simulink library "lib_FaultDetection"  (R2017a)
settings: Solver=VariableStepAuto  StartTime=0.0  StopTime=10.0  RelTol=1e-3
undefined symbols (not defined in the file): cal, ENGTRQ_MSMCH_Degraded_CP, ENGTRQ_MSMCH_ErrCritical_CP, ENGTRQ_MSMCH_LimpHome_CP
libraries: simulink x57, Diagnostic x4, lib_SystemDiag x1
(part 1 of 3)
settings Model: Creator=Di Russo  LastModifiedBy=Di Russo

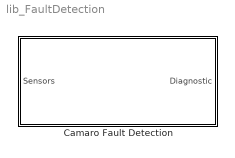
== system lib_FaultDetection ==
  Camaro Fault Detection : Subsystem

== system lib_FaultDetection/Camaro Fault Detection ==
  Sensors : Inport
  Component Diagnostic : Subsystem
  Input Conversions : Subsystem
  Signal Diagnostic : Subsystem
  SystemDiag : lib_SystemDiag/SystemDiag
  Diagnostic : Outport
  wires:
  SystemDiag/1 -> Diagnostic/1
  Sensors/1 -> Input Conversions/1(RawSig)
  Input Conversions/1(VehSig) -> Signal Diagnostic/1(VehSig)
  Component Diagnostic/1(CompDiag) -> SystemDiag/1
  Signal Diagnostic/1(SignalDiag) -> Component Diagnostic/1(SignalDiag)

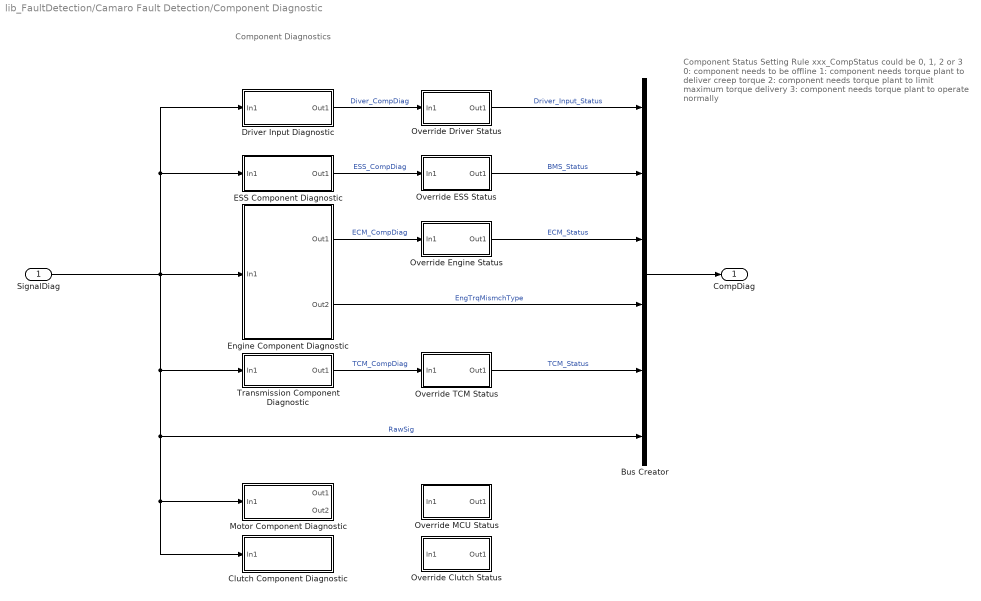
== system lib_FaultDetection/Camaro Fault Detection/Component Diagnostic ==
  note: Component Diagnostics
  note: Component Status Setting Rule
      | xxx_CompStatus could be 0, 1, 2 or 3
      | 0: component needs to be offline
      | 1: component needs torque plant to deliver creep torque
      | 2: component needs torque plant to limit maximum torque delivery
      | 3: component needs torque plant to operate normally
  SignalDiag : Inport
  Bus Creator : BusCreator  Inputs=6
  Clutch Component Diagnostic : Subsystem
  Driver Input Diagnostic : Subsystem
  ESS Component Diagnostic : Subsystem
  Engine Component Diagnostic : Subsystem
  Motor Component Diagnostic : Subsystem
  Override Clutch Status : Subsystem
  Override Driver Status : Subsystem
  Override ESS Status : Subsystem
  Override Engine Status : Subsystem
  Override MCU Status : Subsystem
  Override TCM Status : Subsystem
  Transmission Component Diagnostic : Subsystem
  CompDiag : Outport
  wires:
  Engine Component Diagnostic/2(Out2) -> Bus Creator/4  "EngTrqMismchType"
  Override Driver Status/1(Out1) -> Bus Creator/1  "Driver_Input_Status"
  Override TCM Status/1(Out1) -> Bus Creator/5  "TCM_Status"
  Override Engine Status/1(Out1) -> Bus Creator/3  "ECM_Status"
  Override ESS Status/1(Out1) -> Bus Creator/2  "BMS_Status"
  Transmission Component Diagnostic/1(Out1) -> Override TCM Status/1(In1)  "TCM_CompDiag"
  Engine Component Diagnostic/1(Out1) -> Override Engine Status/1(In1)  "ECM_CompDiag"
  ESS Component Diagnostic/1(Out1) -> Override ESS Status/1(In1)  "ESS_CompDiag"
  Driver Input Diagnostic/1(Out1) -> Override Driver Status/1(In1)  "Diver_CompDiag"
  Bus Creator/1 -> CompDiag/1
  SignalDiag/1 -> Driver Input Diagnostic/1(In1), ESS Component Diagnostic/1(In1), Bus Creator/6, Motor Component Diagnostic/1(In1), Clutch Component Diagnostic/1(In1), Transmission Component Diagnostic/1(In1), Engine Component Diagnostic/1(In1)  "RawSig"

== system lib_FaultDetection/Camaro Fault Detection/Input Conversions ==
  note: These subsystems convert variable types to match those used in the
      | supervisor. In addition, override switches installed on each signal can
      | be used to manually override and signal for testing purposes
  note: Input Conversions and Override Switches
  RawSig : Inport
  BMS_Conversions : Subsystem
  Bus Creator : BusCreator  Inputs=6
  Clutch_Conversions : Subsystem
  DriverInput_Conversions : Subsystem
  ECM_Conversions : Subsystem
  MCU_Conversions : Subsystem
  TCM_Conversions : Subsystem
  VehSig : Outport
  wires:
  TCM_Conversions/1(Out1) -> Bus Creator/4
  ECM_Conversions/1(Out1) -> Bus Creator/3
  RawSig/1 -> Clutch_Conversions/1(Sensors), Bus Creator/6, TCM_Conversions/1(In1), ECM_Conversions/1(In1), BMS_Conversions/1(In1), DriverInput_Conversions/1(In1)  "RawSig"
  BMS_Conversions/1(Out1) -> Bus Creator/2
  Bus Creator/1 -> VehSig/1  "InputConvAndOvrd"
  DriverInput_Conversions/1(Out1) -> Bus Creator/1
  Clutch_Conversions/1(Out1) -> Bus Creator/5

== system lib_FaultDetection/Camaro Fault Detection/Signal Diagnostic ==
  note: Signal Diagnostics
  note: These subsystems evaluate each signal for proper value range and other checks
  VehSig : Inport
  Bus Creator : BusCreator  Inputs=7
  Clutch Signal Diagnostic : Subsystem
  Driver Signal Diagnostic : Subsystem
  ESS Signal Diagnostic : Subsystem
  Engine Signal Diagnostic : Subsystem
  Motor Signal Diagnostic : Subsystem
  Subsystem1 : Subsystem
      mask Display: fprintf('Signal Naming Rule')
  Transmission Signal Diagnostic : Subsystem
  SignalDiag : Outport
  wires:
  Bus Creator/1 -> SignalDiag/1  "SignalDiag"
  Transmission Signal Diagnostic/1(Transmission_SigDiag) -> Bus Creator/5  "Transmission_SigDiag"
  Engine Signal Diagnostic/1(Engine_SigDiag) -> Bus Creator/4  "Engine_SigDiag"
  ESS Signal Diagnostic/1(ESS_SigDiag) -> Bus Creator/2  "ESS_SigDiag"
  Driver Signal Diagnostic/1(Driver_SigDiag) -> Bus Creator/1  "Driver_SigDiag"
  VehSig/1 -> Driver Signal Diagnostic/1(Sensors1), ESS Signal Diagnostic/1(Sensors1), Motor Signal Diagnostic/1(Sensors1), Engine Signal Diagnostic/1(Sensors1), Transmission Signal Diagnostic/1(Sensors1), Bus Creator/7, Clutch Signal Diagnostic/1(Sensors1)
  Clutch Signal Diagnostic/1(Out2) -> Bus Creator/6  "Clutch_SigDiag"
  Motor Signal Diagnostic/1(Motor_SigDiag) -> Bus Creator/3  "Motor_SigDiag"

== system lib_FaultDetection/Camaro Fault Detection/Component Diagnostic/Clutch Component Diagnostic ==
  note: 0: component Offline
      | 1: component Online
  In1 : Inport
  Bus Selector : BusSelector  OutputSignals=Motor_SigDiag.MCURollingAliveActive,Motor_SigDiag.MCUTemp_degC_SigValid,Motor_SigDiag.MotorTemp_degC_SigValid,Motor_SigDiag.Motor_TrqCmd_Nm_SigValid,Motor_SigDiag.Torq_Feedback_Nm_SigValid,Motor_SigDiag.MCUTrqCmd_Nm,Motor_SigDiag.Torq_Feedback_Nm,Motor_SigDiag.Motor_Speed_rpm_SigValid,Motor_SigDiag.MCUTempRange[0_4],Motor_SigDiag.MotorTempRange[0_4],Motor_SigDiag.Direction_Command_SigValid,Motor_SigDiag.Direction_feedback_SigValid,Motor_SigDiag.Inverter_enable_state_SigValid,Motor_SigDiag.Direction_Command_0_1,Motor_SigDiag.Direction_feedback_0_1,Motor_SigDiag.Inverter_enable_state_0_1,Motor_SigDiag.DC_Bus_Voltage_SigValid,Motor_SigDiag.DC_Bus_Voltage_V,ESS_SigDiag.hvBattVolt_V
  wires:
  In1/1 -> Bus Selector/1

== system lib_FaultDetection/Camaro Fault Detection/Component Diagnostic/Driver Input Diagnostic ==
  note: APP1
      | APP2
      | BPP
      | Driver Component Status
      |
      | 1
      | 1
      | 1
      | 1
      |
      | 0
      | 1
      | 1
      | 1
      |
      | 1
      | 0
      | 1
      | 1
      |
      | 0
      | 0
      | 1
      | 0
      |
      | 1
      | 1
      | 0
      | 0
      |
      | 0
      | 0
      | 0
      | 0
  note: Driver_CompStatus
      | 1 = Component Online
      | 0 = Component Offline
  In1 : Inport
  Bus Selector : BusSelector  OutputSignals=Driver_SigDiag.Drv_APP1_[%]_SigValid,Driver_SigDiag.Drv_APP2_[%]_SigValid,Driver_SigDiag.Drv_APP_Agree,Driver_SigDiag.Drv_BPP_[%]_SigValid,Driver_SigDiag.Drv_KeyPos_[0 3]_SigValid,Driver_SigDiag.Drv_PRNDL_SigValid,Driver_SigDiag.Brake_Failed
  Driver_Input_Diag : Stateflow chart  TreatAsAtomicUnit=on
  Logical Operator : Logic  Inputs=3  AllPortsSameDT=off  OutDataTypeStr=boolean
  Out1 : Outport
  wires:
  Bus Selector/7 -> Driver_Input_Diag/5(BrakeFail)  "<Brake_Failed>"
  Bus Selector/6 -> Driver_Input_Diag/4(PRNDL)  "<Drv_PRNDL_SigValid>"
  Bus Selector/5 -> Driver_Input_Diag/3(KeyPos)  "<Drv_KeyPos_[0 3]_SigValid>"
  Bus Selector/3 -> Logical Operator/3  "<Drv_APP_Agree>"
  Logical Operator/1 -> Driver_Input_Diag/1(APP_Valid)  "APP_Valid"
  Driver_Input_Diag/1(Driver_Input_Status) -> Out1/1  "Driver_Input_Status"
  Bus Selector/4 -> Driver_Input_Diag/2(Drv_BPP_SigValid)  "<Drv_BPP_[%]_SigValid>"
  Bus Selector/2 -> Logical Operator/2  "<Drv_APP2_[%]_SigValid>"
  Bus Selector/1 -> Logical Operator/1  "<Drv_APP1_[%]_SigValid>"
  In1/1 -> Bus Selector/1

== system lib_FaultDetection/Camaro Fault Detection/Component Diagnostic/ESS Component Diagnostic ==
  note: (Need modify)
  In1 : Inport
  BMS_CompDiag1 : Stateflow chart  TreatAsAtomicUnit=on
  Bus Selector : BusSelector  OutputSignals=ESS_SigDiag.BMS_RollingAliveActive_SigValid,ESS_SigDiag.BMS_contactorsFailed_Detected,ESS_SigDiag.BMS_essTemp_[degC]_SigValid,ESS_SigDiag.essTempRange[0_4],ESS_SigDiag.BMS_essSOC_0_1_SigValid,ESS_SigDiag.essTempRange[0_4],ESS_SigDiag.essCur_A_SigValid,ESS_SigDiag.BMSgdf_SigValid,Driver_SigDiag.Drv_KeyPos_[0 3]_SigValid
  Compare To Zero : simulink/Logic and Bit Operations/Compare To Zero  relop===  OutDataTypeStr=boolean
  Data Type Conversion : DataTypeConversion
  HVessFltReset : Constant
  Logical Operator : Logic  Operator=OR  AllPortsSameDT=off  OutDataTypeStr=boolean
  Logical Operator1 : Logic  AllPortsSameDT=off  OutDataTypeStr=boolean
  Terminator : Terminator
  Terminator1 : Terminator
  Out1 : Outport
  wires:
  [contactorsFailed_Detected] -> Logical Operator1/1
  Logical Operator1/1 -> BMS_CompDiag1/6(ess_GroundFault)
  Bus Selector/8 -> Logical Operator1/2  "<BMSgdf_SigValid>"
  Logical Operator/1 -> BMS_CompDiag1/7(ClearFault)
  HVessFltReset/1 -> Logical Operator/2
  Compare To Zero/1 -> Logical Operator/1
  Bus Selector/9 -> Compare To Zero/1  "<Drv_KeyPos_[0 3]_SigValid>"
  Bus Selector/7 -> BMS_CompDiag1/5(essCur_A_SigValid)  "<essCur_A_SigValid>"
  Bus Selector/6 -> Terminator1/1  "<essTempRange[0_4]>"
  Bus Selector/5 -> BMS_CompDiag1/4(BMS_essSOC_0_1_SigValid)  "<BMS_essSOC_0_1_SigValid>"
  Data Type Conversion/1 -> BMS_CompDiag1/3(BMS_essTemp_SigValid)  "BMS_essTemp_SigValid"
  Bus Selector/3 -> Data Type Conversion/1  "<BMS_essTemp_[degC]_SigValid>"
  Bus Selector/4 -> Terminator/1  "<essTempRange[0_4]>"
  BMS_CompDiag1/1(BMS_Status) -> Out1/1  "BMS_Status"
  Bus Selector/2 -> BMS_CompDiag1/2(BMS_contactorsFailed_SigValid), [contactorsFailed_Detected]  "<BMS_contactorsFailed_Detected>"
  Bus Selector/1 -> BMS_CompDiag1/1(BMS_RollingAliveActive_SigValid)  "<BMS_RollingAliveActive_SigValid>"
  In1/1 -> Bus Selector/1

== system lib_FaultDetection/Camaro Fault Detection/Component Diagnostic/Engine Component Diagnostic ==
  note: Notes
  note: 0: component needs to be offline
      | 1: component needs torque plant to deliver creep torque
      | 2: component needs torque plant to limit maximum torque delivery
      | 3: component needs torque plant to operate normally
  note: add the temperature, mismatch torquesignal and have different status to the component
  note: Eng_tempRange
      | 1: normal
      | 2: high range
      | 3:above max
  note: ENGTRQ_MSMCH_Degraded_CP (40Nm): ENGTRQ_Degraded fault code.
      | ENGTRQ_MSMCH_LimpHome_CP (70Nm): ENGTRQ_LimpHome
      | ENGTRQ_MSMCH_ErrCritical_CP (100Nm): ENGTRQ_ErrCritical
  note: Eng_Torq_MsmchLevel
      | 1:Normal torque
      | 2: Limit max power
      | 3: Deliver creep torque
      | 4: offline
  In1 : Inport
  Bus Selector : BusSelector  OutputSignals=Engine_SigDiag.ECMRollingAliveActive,Engine_SigDiag.engTrqCmdRecvd_SigValid,Engine_SigDiag.ECMTrqCmd_Nm,Engine_SigDiag.EngActStdyStTorq_Nm,Engine_SigDiag.EngRunAtValid,Engine_SigDiag.Engine_Speed_rpm_SigValid,Engine_SigDiag.Eng_TempValid,Engine_SigDiag.Eng_TempRange[123],Driver_SigDiag.Drv_KeyPos_[0 3]_SigValid
  Bus Selector1 : BusSelector  OutputSignals=Eng_Torque_Mismch_Critical
  Compare To Zero : simulink/Logic and Bit Operations/Compare To Zero  relop===  OutDataTypeStr=boolean
  ECM_CompDiag : Stateflow chart  TreatAsAtomicUnit=on
  Eng_FltReset : Constant
  Eng_Torq_MsmchLevel : Stateflow chart  Commented=on  TreatAsAtomicUnit=on
  Logical Operator : Logic  Operator=OR  AllPortsSameDT=off  OutDataTypeStr=boolean
  Override  engTrqCmd : Subsystem
  Terminator1 : Terminator
  TorqMismatch Detection : Subsystem
  Out1 : Outport
  Out2 : Outport  Port=2
  wires:
  Override  engTrqCmd/1(Out1) -> ECM_CompDiag/2(engTrqCmdRecvd_SigValid)
  Bus Selector1/1 -> ECM_CompDiag/3(Eng_Torq_Msmch)  "<Eng_Torque_Mismch_Critical>"
  TorqMismatch Detection/1(Eng_Torque_Mismch) -> Out2/1, Bus Selector1/1  "EngTrqMismchType"
  Bus Selector/5 -> TorqMismatch Detection/3(In3)  "<EngRunAtValid>"
  Bus Selector/4 -> TorqMismatch Detection/2(In2)  "<EngActStdyStTorq_Nm>"
  Bus Selector/3 -> TorqMismatch Detection/1(In1)  "<ECMTrqCmd_Nm>"
  Bus Selector/8 -> ECM_CompDiag/5(Eng_TempRange_123)  "<Eng_TempRange[123]>"
  Bus Selector/7 -> Terminator1/1  "<Eng_TempValid>"
  Bus Selector/9 -> Compare To Zero/1  "<Drv_KeyPos_[0 3]_SigValid>"
  Logical Operator/1 -> ECM_CompDiag/6(ClearFault)
  Eng_FltReset/1 -> Logical Operator/2
  Compare To Zero/1 -> Logical Operator/1
  ECM_CompDiag/1(ECM_Status) -> Out1/1  "ECM_Status"
  Bus Selector/6 -> ECM_CompDiag/4(Engine_Speed_rpm_SigValid)  "<Engine_Speed_rpm_SigValid>"
  Bus Selector/2 -> Override  engTrqCmd/1(In1)  "<engTrqCmdRecvd_SigValid>"
  Bus Selector/1 -> ECM_CompDiag/1(ECM_RollingAliveActive)  "<ECMRollingAliveActive>"
  In1/1 -> Bus Selector/1

== system lib_FaultDetection/Camaro Fault Detection/Component Diagnostic/Motor Component Diagnostic ==
  note: 0: component needs to be offline
      | 1: component needs torque plant to deliver creep torque
      | 2: component needs torque plant to limit maximum torque delivery
      | 3: component needs torque plant to operate normally
  In1 : Inport
  Bus Creator : BusCreator  Inputs=1
  Bus Selector : BusSelector  OutputSignals=Motor_SigDiag.MCURollingAliveActive,Motor_SigDiag.MCUTemp_degC_SigValid,Motor_SigDiag.MotorTemp_degC_SigValid,Motor_SigDiag.Motor_TrqCmd_Nm_SigValid,Motor_SigDiag.Torq_Feedback_Nm_SigValid,Motor_SigDiag.MCUTrqCmd_Nm,Motor_SigDiag.Torq_Feedback_Nm,Motor_SigDiag.Motor_Speed_rpm_SigValid,Motor_SigDiag.MCUTempRange[0_4],Motor_SigDiag.MotorTempRange[0_4],Motor_SigDiag.Direction_Command_SigValid,Motor_SigDiag.Direction_feedback_SigValid,Motor_SigDiag.Inverter_enable_state_SigValid,Motor_SigDiag.Direction_Command_0_1,Motor_SigDiag.Direction_feedback_0_1,Motor_SigDiag.Inverter_enable_state_0_1,Motor_SigDiag.DC_Bus_Voltage_SigValid,Motor_SigDiag.DC_Bus_Voltage_V,ESS_SigDiag.hvBattVolt_V
  Bus Selector1 : BusSelector  OutputSignals=MCU_Torque_Mismch_Critical
  MCU_CompDiag : Stateflow chart  TreatAsAtomicUnit=on
  MCU_ESS_Voltage_Mismatch : Subsystem
  Motor_Direction_Mismatch : Subsystem
  Override  fault : Subsystem
  Override  fault1 : Subsystem
  Terminator1 : Terminator
  Torque_Mismatch : Subsystem
  Out1 : Outport
  Out2 : Outport  Port=2
  wires:
  In1/1 -> Bus Selector/1
  MCU_CompDiag/1(MCU_Status) -> Bus Creator/1  "MCU_Status"
  Bus Selector/1 -> MCU_CompDiag/1(MCU_RollingAliveActive)  "<MCURollingAliveActive>"
  Bus Selector/2 -> MCU_CompDiag/2(MCUTemp_degC_SigValid)  "<MCUTemp_degC_SigValid>"
  Bus Selector/3 -> MCU_CompDiag/3(MotorTemp_degC_SigValid)  "<MotorTemp_degC_SigValid>"
  Bus Selector/4 -> MCU_CompDiag/4(Motor_TrqCmd_Nm_SigValid)  "<Motor_TrqCmd_Nm_SigValid>"
  Bus Selector/8 -> MCU_CompDiag/7(Motor_Speed_rpm_SigValid)  "<Motor_Speed_rpm_SigValid>"
  Bus Selector/9 -> MCU_CompDiag/8(MCUTempRange)  "<MCUTempRange[0_4]>"
  Bus Creator/1 -> Out1/1
  Bus Selector/13 -> Terminator1/1  "<Inverter_enable_state_SigValid>"
  Bus Selector/6 -> Torque_Mismatch/1(MCU_torq_command)  "<MCUTrqCmd_Nm>"
  Bus Selector/7 -> Torque_Mismatch/2(Torq_feedback)  "<Torq_Feedback_Nm>"
  Bus Selector/14 -> Motor_Direction_Mismatch/1(Direction_Command)  "<Direction_Command_0_1>"
  Bus Selector/15 -> Motor_Direction_Mismatch/2(Direction_Feedback)  "<Direction_feedback_0_1>"
  Bus Selector/16 -> Motor_Direction_Mismatch/3(Inverter_enable_state)  "<Inverter_enable_state_0_1>"
  Bus Selector/11 -> MCU_CompDiag/10(Dir_Command_SigValid)  "<Direction_Command_SigValid>"
  Bus Selector/12 -> MCU_CompDiag/11(Dir_feedback_SigValid)  "<Direction_feedback_SigValid>"
  Bus Selector/5 -> MCU_CompDiag/5(Torq_Feedback_SigValid)  "<Torq_Feedback_Nm_SigValid>"
  Bus Selector/17 -> MCU_CompDiag/13(dc_bus_voltage_SigValid)  "<DC_Bus_Voltage_SigValid>"
  Bus Selector/18 -> MCU_ESS_Voltage_Mismatch/1(MCU_Voltage)  "<DC_Bus_Voltage_V>"
  Bus Selector/19 -> MCU_ESS_Voltage_Mismatch/2(ESS_Voltage)  "< hvBattVolt_V>"
  MCU_ESS_Voltage_Mismatch/1(MCU_ESS_Voltage_Mismch) -> Override  fault/1(In1)
  Motor_Direction_Mismatch/1(Direction_Mismch) -> Override  fault1/1(In1)
  Torque_Mismatch/1(MCU_Torque_Mismch) -> Bus Selector1/1, Out2/1  "MCU_Torque_Mismch"
  Bus Selector1/1 -> MCU_CompDiag/6(MCU_torq_mismch)  "<MCU_Torque_Mismch_Critical>"
  Override  fault/1(Out1) -> MCU_CompDiag/14(Voltage_Mismch)
  Override  fault1/1(Out1) -> MCU_CompDiag/12(Dir_Mismch)
  Bus Selector/10 -> MCU_CompDiag/9(MotTempRange)  "<MotorTempRange[0_4]>"

== system lib_FaultDetection/Camaro Fault Detection/Component Diagnostic/Override Clutch Status ==
  note: Override Switch Subsystem
  note: This subsystem is used to override the model value of a signal to a constant value
  In1 : Inport
  Multiport Switch : MultiPortSwitch  DataPortOrder=Zero-based contiguous  Inputs=2  zeroidx=on
  Override Value : Constant  Value=2  OutDataTypeStr=double
  Signal Override Switch 0 = Use Model 1 = Use Constant : Constant  Value=0
  Out1 : Outport
  wires:
  Override Value/1 -> Multiport Switch/3
  Multiport Switch/1 -> Out1/1
  In1/1 -> Multiport Switch/2
  Signal Override Switch 0 = Use Model 1 = Use Constant/1 -> Multiport Switch/1

== system lib_FaultDetection/Camaro Fault Detection/Component Diagnostic/Override Driver Status ==
  note: Override Switch Subsystem
  note: This subsystem is used to override the model value of a signal to a constant value
  In1 : Inport
  Data Type Conversion3 : DataTypeConversion
  Override Value : Constant  OutDataTypeStr=double
  Override_Driver_Status : Constant  Value=0
  Switch : Switch  Criteria=u2 > Threshold
  Out1 : Outport
  wires:
  Data Type Conversion3/1 -> Switch/3
  Override Value/1 -> Switch/1
  Switch/1 -> Out1/1
  In1/1 -> Data Type Conversion3/1
  Override_Driver_Status/1 -> Switch/2

== system lib_FaultDetection/Camaro Fault Detection/Component Diagnostic/Override ESS Status ==
  note: Override Switch Subsystem
  note: This subsystem is used to override the model value of a signal to a constant value
  In1 : Inport
  Data Type Conversion3 : DataTypeConversion
  Override Value : Constant  Value=2  OutDataTypeStr=double
  Override_ESS_Status : Constant  Value=0
  Switch : Switch  Criteria=u2 > Threshold
  Terminator : Terminator
  Out1 : Outport
  wires:
  Data Type Conversion3/1 -> Switch/3
  Override Value/1 -> Switch/1, Out1/1
  Override_ESS_Status/1 -> Switch/2
  In1/1 -> Data Type Conversion3/1
  Switch/1 -> Terminator/1

== system lib_FaultDetection/Camaro Fault Detection/Component Diagnostic/Override Engine Status ==
  note: Override Switch Subsystem
  note: This subsystem is used to override the model value of a signal to a constant value
  In1 : Inport
  Data Type Conversion3 : DataTypeConversion
  Override Value1 : Constant  Value=2  OutDataTypeStr=double
  Override_Engine_Status : Constant  Value=0
  Switch : Switch  Criteria=u2 > Threshold
  Terminator : Terminator
  Out1 : Outport
  wires:
  Data Type Conversion3/1 -> Switch/3
  Override_Engine_Status/1 -> Switch/2
  Override Value1/1 -> Switch/1, Out1/1
  In1/1 -> Data Type Conversion3/1
  Switch/1 -> Terminator/1

== system lib_FaultDetection/Camaro Fault Detection/Component Diagnostic/Override MCU Status ==
  note: This subsystem is used to override the model value of a signal to a constant value
  note: Override Switch Subsystem
  In1 : Inport
  Multiport Switch : MultiPortSwitch  DataPortOrder=Zero-based contiguous  Inputs=2  zeroidx=on
  Override Value : Constant  Value=2  OutDataTypeStr=double
  Signal Override Switch 0 = Use Model 1 = Use Constant : Constant  Value=0
  Out1 : Outport
  wires:
  Signal Override Switch 0 = Use Model 1 = Use Constant/1 -> Multiport Switch/1
  In1/1 -> Multiport Switch/2
  Multiport Switch/1 -> Out1/1
  Override Value/1 -> Multiport Switch/3

== system lib_FaultDetection/Camaro Fault Detection/Component Diagnostic/Override TCM Status ==
  note: Override Switch Subsystem
  note: This subsystem is used to override the model value of a signal to a constant value
  In1 : Inport
  Data Type Conversion3 : DataTypeConversion
  Override Value1 : Constant  Value=2  OutDataTypeStr=double
  Override_TCM_Status : Constant  Value=0
  Switch : Switch  Criteria=u2 > Threshold
  Out1 : Outport
  wires:
  Data Type Conversion3/1 -> Switch/3
  Override Value1/1 -> Switch/1
  Override_TCM_Status/1 -> Switch/2
  Switch/1 -> Out1/1
  In1/1 -> Data Type Conversion3/1

== system lib_FaultDetection/Camaro Fault Detection/Component Diagnostic/Transmission Component Diagnostic ==
  In1 : Inport
  Bus Selector : BusSelector  OutputSignals=Transmission_SigDiag.TCMRollingAliveActive_SigValid,Transmission_SigDiag.LvrPosTrnsShft_SigValid,Transmission_SigDiag.TransEstGear_SigValid,Transmission_SigDiag.LockupCmd_SigValid,Transmission_SigDiag.VehDirFault
  TCM_CompDia : Stateflow chart  TreatAsAtomicUnit=on
  Out1 : Outport
  wires:
  Bus Selector/5 -> TCM_CompDia/5(VehDirFault)  "<VehDirFault>"
  TCM_CompDia/1(TCM_Status) -> Out1/1  "TCM_Status"
  Bus Selector/4 -> TCM_CompDia/4(LockupCmd_SigValid)  "<LockupCmd_SigValid>"
  Bus Selector/3 -> TCM_CompDia/3(TransEstGear_SigValid)  "<TransEstGear_SigValid>"
  Bus Selector/2 -> TCM_CompDia/2(LvrPosTrnsShft_SigValid)  "<LvrPosTrnsShft_SigValid>"
  Bus Selector/1 -> TCM_CompDia/1(TCMRollingAliveActive_SigValid)  "<TCMRollingAliveActive_SigValid>"
  In1/1 -> Bus Selector/1

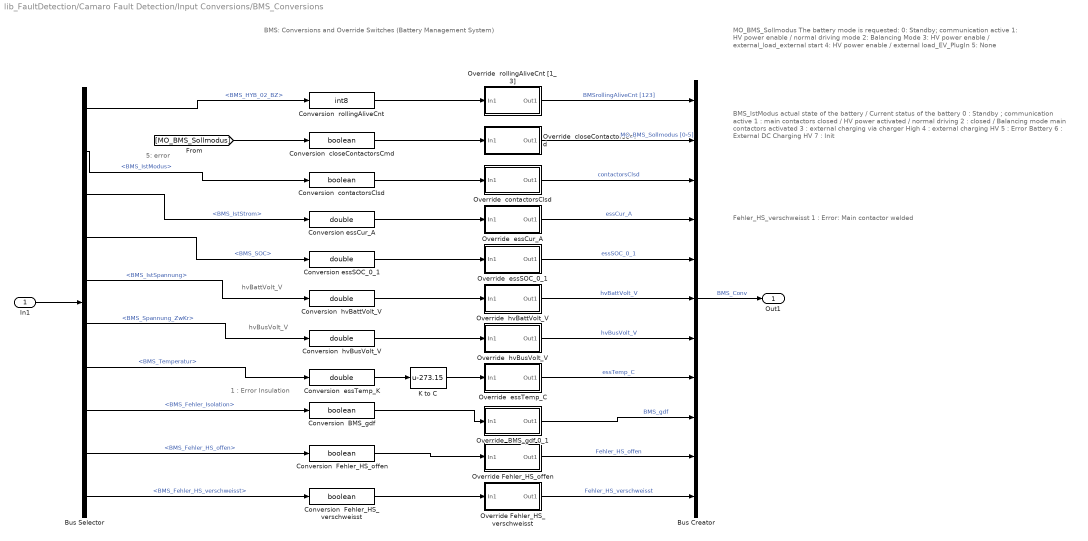
== system lib_FaultDetection/Camaro Fault Detection/Input Conversions/BMS_Conversions ==
  note: BMS: Conversions and Override Switches
      | (Battery Management System)
  note: hvBattVolt_V
  note: hvBusVolt_V
  note: 5: error
  note: 1 : Error Insulation
  note: MO_BMS_Sollmodus
      | The battery mode is requested:
      | 0: Standby; communication active
      | 1: HV power enable / normal driving mode
      | 2: Balancing Mode
      | 3: HV power enable / external_load_external start
      | 4: HV power enable / external load_EV_PlugIn
      | 5: None
  note: BMS_IstModus
      | actual state of the battery / Current status of the battery
      | 0 : Standby ; communication active
      | 1 : main contactors closed / HV power activated / normal driving
      | 2 : closed / Balancing mode main contactors activated
      | 3 : external charging via charger High
      | 4 : external charging HV
      | 5 : Error Battery
      | 6 : External DC Charging HV
      | 7 : Init
  note: Fehler_HS_verschweisst
      | 1 : Error: Main contactor welded
  In1 : Inport
  Bus Creator : BusCreator  Inputs=11
  Bus Selector : BusSelector  OutputSignals=from_CAN.fromHV_CAN.from_BMSHybrid.BMS_HYB_02.BMS_HYB_02_BZ,from_CAN.fromHV_CAN.from_BMSHybrid.BMS_HYB_02.BMS_IstModus,from_CAN.fromHV_CAN.from_BMSHybrid.BMS_HYB_02.BMS_IstStrom,from_CAN.fromHV_CAN.from_BMSHybrid.BMS_SOC,from_CAN.fromHV_CAN.from_BMSHybrid.BMS_HYB_02.BMS_IstSpannung,from_CAN.fromHV_CAN.from_BMSHybrid.BMS_Spannung_ZwKr,from_CAN.fromHV_CAN.from_BMSHybrid.BMS_Temperatur,from_CAN.fromHV_CAN.from_BMSHybrid.BMS_Fehler_Isolation,from_CAN.fromHV_CAN.from_BMSHybrid.BMS_HYB_02.BMS_Fehler_HS_offen,from_CAN.fromHV_CAN.from_BMSHybrid.BMS_Fehler_HS_verschweisst
  Conversion  BMS_gdf : DataTypeConversion  OutDataTypeStr=boolean
  Conversion  Fehler_HS_offen : DataTypeConversion  OutDataTypeStr=boolean
  Conversion  Fehler_HS_verschweisst : DataTypeConversion  OutDataTypeStr=boolean
  Conversion  closeContactorsCmd : DataTypeConversion  OutDataTypeStr=boolean
  Conversion  contactorsClsd : DataTypeConversion  OutDataTypeStr=boolean
  Conversion  essTemp_K : DataTypeConversion  OutDataTypeStr=double
  Conversion  hvBattVolt_V : DataTypeConversion  OutDataTypeStr=double
  Conversion  hvBusVolt_V : DataTypeConversion  OutDataTypeStr=double
  Conversion  rollingAliveCnt : DataTypeConversion  OutDataTypeStr=int8
  Conversion essCur_A : DataTypeConversion  OutDataTypeStr=double
  Conversion essSOC_0_1 : DataTypeConversion  OutDataTypeStr=double
  K to C : Bias  Bias=-273.15
  Override  BMS_gdf 0_1 : Subsystem
  Override  closeContactorsCmd : Subsystem
  Override  contactorsClsd : Subsystem
  Override  essCur_A : Subsystem
  Override  essSOC_0_1 : Subsystem
  Override  essTemp_C : Subsystem
  Override  hvBattVolt_V : Subsystem
  Override  hvBusVolt_V : Subsystem
  Override  rollingAliveCnt [1_3] : Subsystem
  Override Fehler_HS_offen : Subsystem
  Override Fehler_HS_verschweisst : Subsystem
  Out1 : Outport
  wires:
  Override Fehler_HS_verschweisst/1(Out1) -> Bus Creator/11  "Fehler_HS_verschweisst"
  Conversion  Fehler_HS_verschweisst/1 -> Override Fehler_HS_verschweisst/1(In1)
  Bus Selector/10 -> Conversion  Fehler_HS_verschweisst/1  "<BMS_Fehler_HS_verschweisst>"
  Override Fehler_HS_offen/1(Out1) -> Bus Creator/10  "Fehler_HS_offen"
  Conversion  Fehler_HS_offen/1 -> Override Fehler_HS_offen/1(In1)
  Bus Selector/9 -> Conversion  Fehler_HS_offen/1  "<BMS_Fehler_HS_offen>"
  [MO_BMS_Sollmodus] -> Conversion  closeContactorsCmd/1
  Bus Selector/6 -> Conversion  hvBusVolt_V/1  "<BMS_Spannung_ZwKr>"
  Bus Selector/1 -> Conversion  rollingAliveCnt/1  "<BMS_HYB_02_BZ>"
  Bus Selector/3 -> Conversion essCur_A/1  "<BMS_IstStrom>"
  Bus Selector/4 -> Conversion essSOC_0_1/1  "<BMS_SOC>"
  Bus Selector/5 -> Conversion  hvBattVolt_V/1  "<BMS_IstSpannung>"
  Bus Selector/8 -> Conversion  BMS_gdf/1  "<BMS_Fehler_Isolation>"
  Bus Selector/7 -> Conversion  essTemp_K/1  "<BMS_Temperatur>"
  Bus Selector/2 -> Conversion  contactorsClsd/1  "<BMS_IstModus>"
  Override  BMS_gdf 0_1/1(Out1) -> Bus Creator/9  "BMS_gdf"
  Conversion  BMS_gdf/1 -> Override  BMS_gdf 0_1/1(In1)
  K to C/1 -> Override  essTemp_C/1(In1)
  Override  essTemp_C/1(Out1) -> Bus Creator/8  "essTemp_C"
  Conversion  essTemp_K/1 -> K to C/1
  Override  hvBusVolt_V/1(Out1) -> Bus Creator/7  "hvBusVolt_V"
  Override  essCur_A/1(Out1) -> Bus Creator/4  "essCur_A"
  Override  hvBattVolt_V/1(Out1) -> Bus Creator/6  "hvBattVolt_V"
  Override  essSOC_0_1/1(Out1) -> Bus Creator/5  "essSOC_0_1"
  Override  contactorsClsd/1(Out1) -> Bus Creator/3  "contactorsClsd"
  Conversion  hvBusVolt_V/1 -> Override  hvBusVolt_V/1(In1)
  Conversion  hvBattVolt_V/1 -> Override  hvBattVolt_V/1(In1)
  Conversion essSOC_0_1/1 -> Override  essSOC_0_1/1(In1)
  Conversion essCur_A/1 -> Override  essCur_A/1(In1)
  Conversion  contactorsClsd/1 -> Override  contactorsClsd/1(In1)
  Override  closeContactorsCmd/1(Out1) -> Bus Creator/2  "MO_BMS_Sollmodus [0-5]"
  Conversion  closeContactorsCmd/1 -> Override  closeContactorsCmd/1(In1)
  Bus Creator/1 -> Out1/1  "BMS_Conv"
  Override  rollingAliveCnt [1_3]/1(Out1) -> Bus Creator/1  "BMSrollingAliveCnt [123]"
  Conversion  rollingAliveCnt/1 -> Override  rollingAliveCnt [1_3]/1(In1)
  In1/1 -> Bus Selector/1

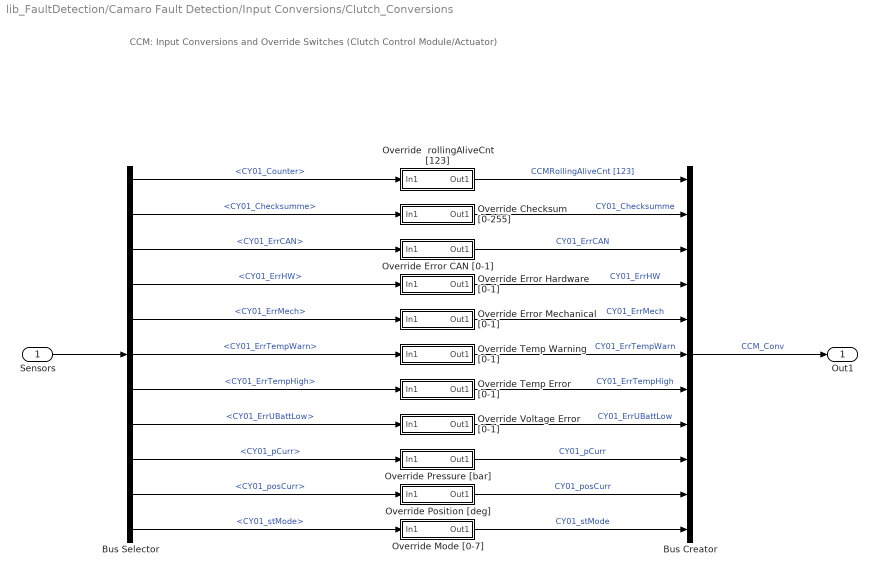
== system lib_FaultDetection/Camaro Fault Detection/Input Conversions/Clutch_Conversions ==
  note: CCM: Input Conversions and Override Switches
      | (Clutch Control Module/Actuator)
  Sensors : Inport
  Bus Creator : BusCreator  Inputs=11
  Bus Selector : BusSelector  OutputSignals=from_CAN.fromEBCAN.from_CCU.CY01_Counter,from_CAN.fromEBCAN.from_CCU.CY01_Checksumme,from_CAN.fromEBCAN.from_CCU.CY01_ErrCAN,from_CAN.fromEBCAN.from_CCU.CY01_ErrHW,from_CAN.fromEBCAN.from_CCU.CY01_ErrMech,from_CAN.fromEBCAN.from_CCU.CY01_ErrTempWarn,from_CAN.fromEBCAN.from_CCU.CY01_ErrTempHigh,from_CAN.fromEBCAN.from_CCU.CY01_ErrUBattLow,from_CAN.fromEBCAN.from_CCU.CY01_pCurr,from_CAN.fromEBCAN.from_CCU.CY01_posCurr,from_CAN.fromEBCAN.from_CCU.CY01_stMode
  Override  rollingAliveCnt [123] : Subsystem
  Override Checksum [0-255] : Subsystem
  Override Error CAN [0-1] : Subsystem
  Override Error Hardware [0-1] : Subsystem
  Override Error Mechanical [0-1] : Subsystem
  Override Mode [0-7] : Subsystem
  Override Position [deg] : Subsystem
  Override Pressure [bar] : Subsystem
  Override Temp Error [0-1] : Subsystem
  Override Temp Warning [0-1] : Subsystem
  Override Voltage Error [0-1] : Subsystem
  Out1 : Outport
  wires:
  Bus Creator/1 -> Out1/1  "CCM_Conv"
  Override  rollingAliveCnt [123]/1(Out1) -> Bus Creator/1  "CCMRollingAliveCnt [123]"
  Bus Selector/1 -> Override  rollingAliveCnt [123]/1(In1)  "<CY01_Counter>"
  Sensors/1 -> Bus Selector/1
  Bus Selector/2 -> Override Checksum [0-255]/1(In1)  "<CY01_Checksumme>"
  Bus Selector/3 -> Override Error CAN [0-1]/1(In1)  "<CY01_ErrCAN>"
  Bus Selector/4 -> Override Error Hardware [0-1]/1(In1)  "<CY01_ErrHW>"
  Bus Selector/5 -> Override Error Mechanical [0-1]/1(In1)  "<CY01_ErrMech>"
  Bus Selector/6 -> Override Temp Warning [0-1]/1(In1)  "<CY01_ErrTempWarn>"
  Bus Selector/7 -> Override Temp Error [0-1]/1(In1)  "<CY01_ErrTempHigh>"
  Bus Selector/8 -> Override Voltage Error [0-1]/1(In1)  "<CY01_ErrUBattLow>"
  Override Checksum [0-255]/1(Out1) -> Bus Creator/2  "CY01_Checksumme"
  Override Error CAN [0-1]/1(Out1) -> Bus Creator/3  "CY01_ErrCAN"
  Override Error Hardware [0-1]/1(Out1) -> Bus Creator/4  "CY01_ErrHW"
  Override Error Mechanical [0-1]/1(Out1) -> Bus Creator/5  "CY01_ErrMech"
  Override Temp Warning [0-1]/1(Out1) -> Bus Creator/6  "CY01_ErrTempWarn"
  Override Temp Error [0-1]/1(Out1) -> Bus Creator/7  "CY01_ErrTempHigh"
  Override Voltage Error [0-1]/1(Out1) -> Bus Creator/8  "CY01_ErrUBattLow"
  Bus Selector/9 -> Override Pressure [bar]/1(In1)  "<CY01_pCurr>"
  Bus Selector/10 -> Override Position [deg]/1(In1)  "<CY01_posCurr>"
  Bus Selector/11 -> Override Mode [0-7]/1(In1)  "<CY01_stMode>"
  Override Pressure [bar]/1(Out1) -> Bus Creator/9  "CY01_pCurr"
  Override Position [deg]/1(Out1) -> Bus Creator/10  "CY01_posCurr"
  Override Mode [0-7]/1(Out1) -> Bus Creator/11  "CY01_stMode"

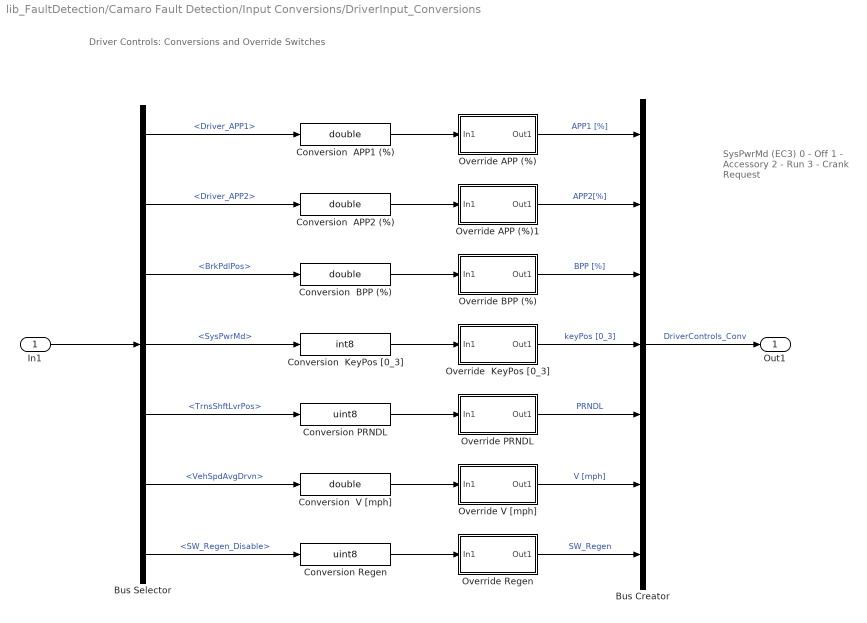
== system lib_FaultDetection/Camaro Fault Detection/Input Conversions/DriverInput_Conversions ==
  note: Driver Controls: Conversions and Override Switches
  note: SysPwrMd (EC3)
      | 0 - Off
      | 1 -  Accessory
      | 2 - Run
      | 3 - Crank Request
  In1 : Inport
  Bus Creator : BusCreator  Inputs=7
  Bus Selector : BusSelector  OutputSignals=from_Analog.Driver_APP1,from_Analog.Driver_APP2,from_CAN.fromVEH_CAN.from_BCM.BrkPdlPos,from_CAN.fromVEH_CAN.from_BCM.SysPwrMd,from_CAN.fromVEH_CAN.from_TCM.TrnsShftLvrPos,from_CAN.fromEBCAN.from_ECM.VehSpdAvgDrvn,from_Digital.SW_Regen_Disable
  Conversion  APP1 (%) : DataTypeConversion  OutDataTypeStr=double
  Conversion  APP2 (%) : DataTypeConversion  OutDataTypeStr=double
  Conversion  BPP (%) : DataTypeConversion  OutDataTypeStr=double
  Conversion  KeyPos [0_3] : DataTypeConversion  OutDataTypeStr=int8
  Conversion  V [mph] : DataTypeConversion  OutDataTypeStr=double
  Conversion PRNDL : DataTypeConversion  OutDataTypeStr=uint8
  Conversion Regen : DataTypeConversion  OutDataTypeStr=uint8
  Override  KeyPos [0_3] : Subsystem
  Override APP (%) : Subsystem
  Override APP (%)1 : Subsystem
  Override BPP (%) : Subsystem
  Override PRNDL : Subsystem
  Override Regen : Subsystem
  Override V [mph] : Subsystem
  Out1 : Outport
  wires:
  Override Regen/1(Out1) -> Bus Creator/7  "SW_Regen"
  Conversion Regen/1 -> Override Regen/1(In1)
  Bus Selector/7 -> Conversion Regen/1  "<SW_Regen_Disable>"
  Override V [mph]/1(Out1) -> Bus Creator/6  "V [mph]"
  Conversion  V [mph]/1 -> Override V [mph]/1(In1)
  Bus Selector/6 -> Conversion  V [mph]/1  "<VehSpdAvgDrvn>"
  Conversion  APP2 (%)/1 -> Override APP (%)1/1(In1)
  Override APP (%)1/1(Out1) -> Bus Creator/2  "APP2[%]"
  Bus Selector/5 -> Conversion PRNDL/1  "<TrnsShftLvrPos>"
  Bus Selector/2 -> Conversion  APP2 (%)/1  "<Driver_APP2>"
  Override PRNDL/1(Out1) -> Bus Creator/5  "PRNDL"
  Conversion PRNDL/1 -> Override PRNDL/1(In1)
  Conversion  BPP (%)/1 -> Override BPP (%)/1(In1)
  Bus Creator/1 -> Out1/1  "DriverControls_Conv"
  Override  KeyPos [0_3]/1(Out1) -> Bus Creator/4  "keyPos [0_3]"
  Override BPP (%)/1(Out1) -> Bus Creator/3  "BPP [%]"
  Conversion  KeyPos [0_3]/1 -> Override  KeyPos [0_3]/1(In1)
  Bus Selector/4 -> Conversion  KeyPos [0_3]/1  "<SysPwrMd>"
  Bus Selector/3 -> Conversion  BPP (%)/1  "<BrkPdlPos>"
  Bus Selector/1 -> Conversion  APP1 (%)/1  "<Driver_APP1>"
  Override APP (%)/1(Out1) -> Bus Creator/1  "APP1 [%]"
  Conversion  APP1 (%)/1 -> Override APP (%)/1(In1)
  In1/1 -> Bus Selector/1

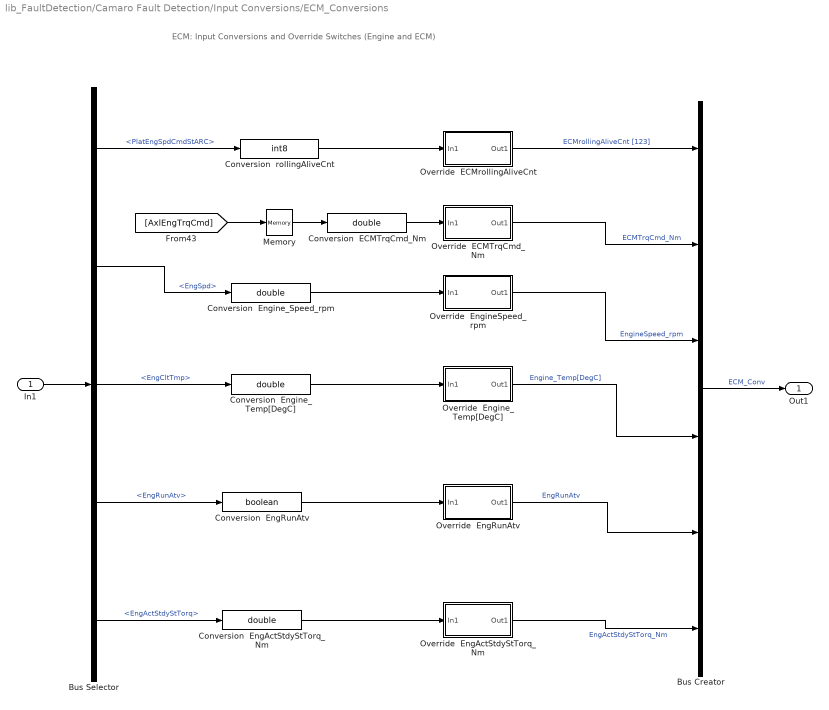
== system lib_FaultDetection/Camaro Fault Detection/Input Conversions/ECM_Conversions ==
  note: ECM: Input Conversions and Override Switches
      | (Engine and ECM)
  In1 : Inport
  Bus Creator : BusCreator  Inputs=6
  Bus Selector : BusSelector  OutputSignals=from_CAN.fromEBCAN.from_ECM.PlatEngSpdCmdStARC,from_CAN.fromEBCAN.from_ECM.EngSpd,from_CAN.fromEBCAN.from_ECM.EngCltTmp,from_CAN.fromEBCAN.from_ECM.EngRunAtv,from_CAN.fromEBCAN.from_ECM.EngActStdyStTorq
  Conversion  ECMTrqCmd_Nm : DataTypeConversion  OutDataTypeStr=double
  Conversion  EngActStdyStTorq_Nm : DataTypeConversion  OutDataTypeStr=double
  Conversion  EngRunAtv : DataTypeConversion  OutDataTypeStr=boolean
  Conversion  Engine_Speed_rpm : DataTypeConversion  OutDataTypeStr=double
  Conversion  Engine_Temp[DegC] : DataTypeConversion  OutDataTypeStr=double
  Conversion  rollingAliveCnt : DataTypeConversion  OutDataTypeStr=int8
  Memory : Memory
  Override  ECMTrqCmd_Nm : Subsystem
  Override  ECMrollingAliveCnt : Subsystem
  Override  EngActStdyStTorq_Nm : Subsystem
  Override  EngRunAtv : Subsystem
  Override  EngineSpeed_rpm : Subsystem
  Override  Engine_Temp[DegC] : Subsystem
  Out1 : Outport
  wires:
  Memory/1 -> Conversion  ECMTrqCmd_Nm/1
  [AxlEngTrqCmd] -> Memory/1
  Bus Selector/1 -> Conversion  rollingAliveCnt/1  "<PlatEngSpdCmdStARC>"
  Override  EngActStdyStTorq_Nm/1(Out1) -> Bus Creator/6  "EngActStdyStTorq_Nm"
  Override  EngRunAtv/1(Out1) -> Bus Creator/5  "EngRunAtv"
  Override  Engine_Temp[DegC]/1(Out1) -> Bus Creator/4  "Engine_Temp[DegC]"
  Conversion  EngActStdyStTorq_Nm/1 -> Override  EngActStdyStTorq_Nm/1(In1)
  Conversion  EngRunAtv/1 -> Override  EngRunAtv/1(In1)
  Conversion  Engine_Temp[DegC]/1 -> Override  Engine_Temp[DegC]/1(In1)
  Bus Selector/5 -> Conversion  EngActStdyStTorq_Nm/1  "<EngActStdyStTorq>"
  Bus Selector/4 -> Conversion  EngRunAtv/1  "<EngRunAtv>"
  Bus Selector/3 -> Conversion  Engine_Temp[DegC]/1  "<EngCltTmp>"
  Override  EngineSpeed_rpm/1(Out1) -> Bus Creator/3  "EngineSpeed_rpm"
  Conversion  Engine_Speed_rpm/1 -> Override  EngineSpeed_rpm/1(In1)
  Bus Selector/2 -> Conversion  Engine_Speed_rpm/1  "<EngSpd>"
  Conversion  ECMTrqCmd_Nm/1 -> Override  ECMTrqCmd_Nm/1(In1)
  Override  ECMTrqCmd_Nm/1(Out1) -> Bus Creator/2  "ECMTrqCmd_Nm"
  Bus Creator/1 -> Out1/1  "ECM_Conv"
  Override  ECMrollingAliveCnt/1(Out1) -> Bus Creator/1  "ECMrollingAliveCnt [123]"
  Conversion  rollingAliveCnt/1 -> Override  ECMrollingAliveCnt/1(In1)
  In1/1 -> Bus Selector/1

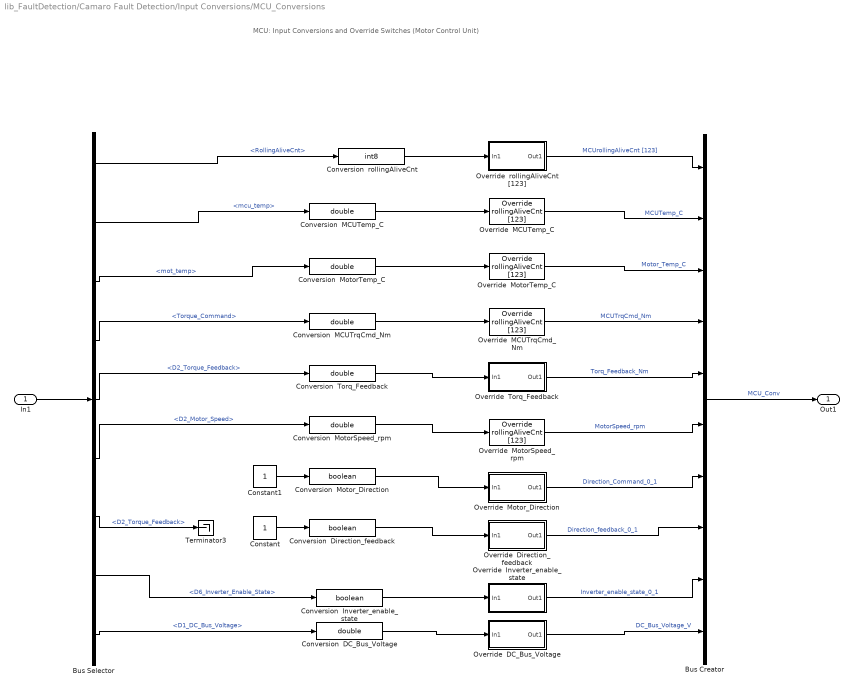
== system lib_FaultDetection/Camaro Fault Detection/Input Conversions/MCU_Conversions ==
  note: MCU: Input Conversions and Override Switches
      | (Motor Control Unit)
  In1 : Inport
  Bus Creator : BusCreator  Inputs=10
  Bus Selector : BusSelector  OutputSignals=from_CAN.fromHV_CAN.from_MCU.RollingAliveCnt,from_CAN.fromHV_CAN.from_MCU.mcu_temp,from_CAN.fromHV_CAN.from_MCU.mot_temp,from_CAN.fromHV_CAN.from_MCU.Torque_Command,from_CAN.fromHV_CAN.from_MCU.D2_Torque_Feedback,from_CAN.fromHV_CAN.from_MCU.D2_Motor_Speed,from_CAN.fromHV_CAN.from_MCU.D2_Torque_Feedback,from_CAN.fromHV_CAN.from_MCU.D6_Inverter_Enable_State,from_CAN.fromHV_CAN.from_MCU.D1_DC_Bus_Voltage
  Constant : Constant
  Constant1 : Constant
  Conversion  DC_Bus_Voltage : DataTypeConversion  OutDataTypeStr=double
  Conversion  Direction_feedback : DataTypeConversion  OutDataTypeStr=boolean
  Conversion  Inverter_enable_state : DataTypeConversion  OutDataTypeStr=boolean
  Conversion  MCUTemp_C : DataTypeConversion  OutDataTypeStr=double
  Conversion  MCUTrqCmd_Nm : DataTypeConversion  OutDataTypeStr=double
  Conversion  MotorSpeed_rpm : DataTypeConversion  OutDataTypeStr=double
  Conversion  MotorTemp_C : DataTypeConversion  OutDataTypeStr=double
  Conversion  Motor_Direction : DataTypeConversion  OutDataTypeStr=boolean
  Conversion  Torq_Feedback : DataTypeConversion  OutDataTypeStr=double
  Conversion  rollingAliveCnt : DataTypeConversion  OutDataTypeStr=int8
  Override  DC_Bus_Voltage : Subsystem
  Override  Direction_feedback : Subsystem
  Override  Inverter_enable_state : Subsystem
  "Override  MCUTemp_C " : Diagnostic/Camaro Diagnostic/Input Conversions/MCU_Conversions/Override  rollingAliveCnt [123]
  Override  MCUTrqCmd_Nm : Diagnostic/Camaro Diagnostic/Input Conversions/MCU_Conversions/Override  rollingAliveCnt [123]
  Override  MotorSpeed_rpm : Diagnostic/Camaro Diagnostic/Input Conversions/MCU_Conversions/Override  rollingAliveCnt [123]
  Override  MotorTemp_C : Diagnostic/Camaro Diagnostic/Input Conversions/MCU_Conversions/Override  rollingAliveCnt [123]
  Override  Motor_Direction : Subsystem
  Override  Torq_Feedback : Subsystem
  Override  rollingAliveCnt [123] : Subsystem
  Terminator3 : Terminator
  Out1 : Outport
  wires:
  In1/1 -> Bus Selector/1
  Conversion  rollingAliveCnt/1 -> Override  rollingAliveCnt [123]/1(In1)
  Override  rollingAliveCnt [123]/1(Out1) -> Bus Creator/1  "MCUrollingAliveCnt [123]"
  Bus Creator/1 -> Out1/1  "MCU_Conv"
  "Override  MCUTemp_C "/1 -> Bus Creator/2  "MCUTemp_C"
  Conversion  MCUTemp_C/1 -> "Override  MCUTemp_C "/1
  Bus Selector/3 -> Conversion  MotorTemp_C/1  "<mot_temp>"
  Conversion  MotorTemp_C/1 -> Override  MotorTemp_C/1
  Override  MotorTemp_C/1 -> Bus Creator/3  "Motor_Temp_C"
  Bus Selector/4 -> Conversion  MCUTrqCmd_Nm/1  "<Torque_Command>"
  Conversion  MCUTrqCmd_Nm/1 -> Override  MCUTrqCmd_Nm/1
  Override  MCUTrqCmd_Nm/1 -> Bus Creator/4  "MCUTrqCmd_Nm"
  Bus Selector/6 -> Conversion  MotorSpeed_rpm/1  "<D2_Motor_Speed>"
  Conversion  MotorSpeed_rpm/1 -> Override  MotorSpeed_rpm/1
  Override  MotorSpeed_rpm/1 -> Bus Creator/6  "MotorSpeed_rpm"
  Bus Selector/5 -> Conversion  Torq_Feedback/1  "<D2_Torque_Feedback>"
  Conversion  Torq_Feedback/1 -> Override  Torq_Feedback/1(In1)
  Override  Torq_Feedback/1(Out1) -> Bus Creator/5  "Torq_Feedback_Nm"
  Conversion  Motor_Direction/1 -> Override  Motor_Direction/1(In1)
  Override  Motor_Direction/1(Out1) -> Bus Creator/7  "Direction_Command_0_1"
  Bus Selector/8 -> Conversion  Inverter_enable_state/1  "<D6_Inverter_Enable_State>"
  Conversion  Direction_feedback/1 -> Override  Direction_feedback/1(In1)
  Conversion  Inverter_enable_state/1 -> Override  Inverter_enable_state/1(In1)
  Override  Direction_feedback/1(Out1) -> Bus Creator/8  "Direction_feedback_0_1"
  Override  Inverter_enable_state/1(Out1) -> Bus Creator/9  "Inverter_enable_state_0_1"
  Bus Selector/9 -> Conversion  DC_Bus_Voltage/1  "<D1_DC_Bus_Voltage>"
  Conversion  DC_Bus_Voltage/1 -> Override  DC_Bus_Voltage/1(In1)
  Override  DC_Bus_Voltage/1(Out1) -> Bus Creator/10  "DC_Bus_Voltage_V"
  Constant/1 -> Conversion  Direction_feedback/1
  Constant1/1 -> Conversion  Motor_Direction/1
  Bus Selector/1 -> Conversion  rollingAliveCnt/1  "<RollingAliveCnt>"
  Bus Selector/2 -> Conversion  MCUTemp_C/1  "<mcu_temp>"
  Bus Selector/7 -> Terminator3/1  "<D2_Torque_Feedback>"

== system lib_FaultDetection/Camaro Fault Detection/Input Conversions/TCM_Conversions ==
  note: TCM: Input Conversions and Override Switches
      | (Transmission Control Module)
  In1 : Inport
  Bus Creator : BusCreator  Inputs=4
  Bus Selector : BusSelector  OutputSignals=from_CAN.fromVEH_CAN.from_TCM.TrnsShftLvrPos,from_CAN.fromVEH_CAN.from_TCM.TransEstGear,from_CAN.fromVEH_CAN.from_TCM.TrnsTrqCnvCltCmndMd
  Conversion  LockupCmd : DataTypeConversion  OutDataTypeStr=boolean
  Conversion  LvrPosTrnsShft : DataTypeConversion  OutDataTypeStr=int8
  Conversion  TransEstGear : DataTypeConversion  OutDataTypeStr=int8
  Conversion  rollingAliveCnt : DataTypeConversion  OutDataTypeStr=int8
  Override  LockupCmd : Subsystem
  "Override  LvrPosTrnsShft " : Subsystem
  Override  TransEstGear : Subsystem
  Override  rollingAliveCnt [123] : Subsystem
  TCM_RollinAliveCounter : Subsystem
  Out1 : Outport
  wires:
  TCM_RollinAliveCounter/1(Out1) -> Conversion  rollingAliveCnt/1
  In1/1 -> Bus Selector/1
  Conversion  rollingAliveCnt/1 -> Override  rollingAliveCnt [123]/1(In1)
  Override  rollingAliveCnt [123]/1(Out1) -> Bus Creator/1  "TCMrollingAliveCnt [123]"
  Bus Creator/1 -> Out1/1  "TCM_Conv"
  Bus Selector/1 -> Conversion  LvrPosTrnsShft/1  "<TrnsShftLvrPos>"
  "Override  LvrPosTrnsShft "/1(Out1) -> Bus Creator/2  "LvrPosTrnsShft"
  Conversion  LvrPosTrnsShft/1 -> "Override  LvrPosTrnsShft "/1(In1)
  Bus Selector/2 -> Conversion  TransEstGear/1  "<TransEstGear>"
  Conversion  TransEstGear/1 -> Override  TransEstGear/1(In1)
  Override  TransEstGear/1(Out1) -> Bus Creator/3  "TransEstGear"
  Bus Selector/3 -> Conversion  LockupCmd/1  "<TrnsTrqCnvCltCmndMd>"
  Conversion  LockupCmd/1 -> Override  LockupCmd/1(In1)
  Override  LockupCmd/1(Out1) -> Bus Creator/4  "LockupCmd_0_1"

== system lib_FaultDetection/Camaro Fault Detection/Signal Diagnostic/Clutch Signal Diagnostic ==
  note: CCM : Signal Diagnostic
  Sensors1 : Inport
  Bus Creator : BusCreator  Inputs=10
  Bus Selector : BusSelector  OutputSignals=CCM_Conv.CCMRollingAliveCnt [123],CCM_Conv.CY01_ErrCAN,CCM_Conv.CY01_ErrHW,CCM_Conv.CY01_ErrMech,CCM_Conv.CY01_ErrTempWarn,CCM_Conv.CY01_ErrTempHigh,CCM_Conv.CY01_ErrUBattLow,CCM_Conv.CY01_pCurr,CCM_Conv.CY01_posCurr,CCM_Conv.CY01_stMode
  CAN Error Flag Active? : simulink/Logic and Bit Operations/Compare To Constant  relop===  const=0  OutDataTypeStr=boolean
  HW Error Flag Active? : simulink/Logic and Bit Operations/Compare To Constant  relop===  const=0  OutDataTypeStr=boolean
  Mech Error Flag Active? : simulink/Logic and Bit Operations/Compare To Constant  relop===  const=0  OutDataTypeStr=boolean
  Mode Interval Test : simulink/Logic and Bit Operations/Interval Test  IntervalClosedRight=on  uplimit=7  IntervalClosedLeft=on  lowlimit=0  OutDataTypeStr=boolean
  Position Interval Test : simulink/Logic and Bit Operations/Interval Test  IntervalClosedRight=on  uplimit=8190  IntervalClosedLeft=on  lowlimit=0  OutDataTypeStr=boolean
  Pressure Interval Test : simulink/Logic and Bit Operations/Interval Test  IntervalClosedRight=on  uplimit=50.6  IntervalClosedLeft=on  lowlimit=0  OutDataTypeStr=boolean
  Rolling Alive Counter Detection : Subsystem
  Temp Error Flag Active? : simulink/Logic and Bit Operations/Compare To Constant  relop===  const=1  OutDataTypeStr=boolean
  Temp Warning Flag Active? : simulink/Logic and Bit Operations/Compare To Constant  relop===  const=1  OutDataTypeStr=boolean
  Voltage Error Flag Active? : simulink/Logic and Bit Operations/Compare To Constant  relop===  const=1  OutDataTypeStr=boolean
  Out2 : Outport
  wires:
  Sensors1/1 -> Bus Selector/1
  Bus Creator/1 -> Out2/1
  Bus Selector/1 -> Rolling Alive Counter Detection/1(In1)  "<CCMRollingAliveCnt [123]>"
  Rolling Alive Counter Detection/1(Out1) -> Bus Creator/1  "CCM_RollingAliveActive_SigValid"
  Bus Selector/2 -> CAN Error Flag Active?/1  "<CY01_ErrCAN>"
  CAN Error Flag Active?/1 -> Bus Creator/2  "CCM_CANTransmission_Valid"
  Bus Selector/3 -> HW Error Flag Active?/1  "<CY01_ErrHW>"
  HW Error Flag Active?/1 -> Bus Creator/3  "CCM_HardwareStatus_Valid"
  Bus Selector/4 -> Mech Error Flag Active?/1  "<CY01_ErrMech>"
  Mech Error Flag Active?/1 -> Bus Creator/4  "CCM_MechStatus_Valid"
  Bus Selector/5 -> Temp Warning Flag Active?/1  "<CY01_ErrTempWarn>"
  Temp Warning Flag Active?/1 -> Bus Creator/5  "CCM_WarnTemp"
  Bus Selector/6 -> Temp Error Flag Active?/1  "<CY01_ErrTempHigh>"
  Temp Error Flag Active?/1 -> Bus Creator/6  "CCM_ErrTemp"
  Bus Selector/7 -> Voltage Error Flag Active?/1  "<CY01_ErrUBattLow>"
  Voltage Error Flag Active?/1 -> Bus Creator/7  "CCM_ErrVoltage"
  Bus Selector/8 -> Pressure Interval Test/1  "<CY01_pCurr>"
  Pressure Interval Test/1 -> Bus Creator/8  "CCM_PistPressValid"
  Bus Selector/9 -> Position Interval Test/1  "<CY01_posCurr>"
  Position Interval Test/1 -> Bus Creator/9  "CCM_PistPosValid"
  Bus Selector/10 -> Mode Interval Test/1  "<CY01_stMode>"
  Mode Interval Test/1 -> Bus Creator/10  "CCM_ModeValid"

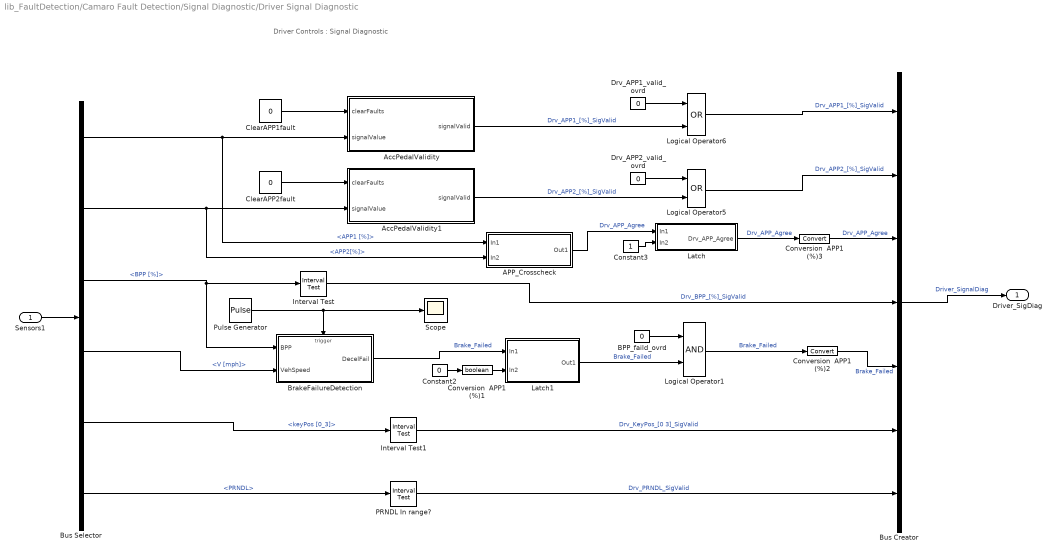
== system lib_FaultDetection/Camaro Fault Detection/Signal Diagnostic/Driver Signal Diagnostic ==
  note: Driver Controls : Signal Diagnostic
  Sensors1 : Inport
  APP_Crosscheck : Subsystem
  AccPedalValidity : Stateflow chart  TreatAsAtomicUnit=on
  AccPedalValidity1 : Stateflow chart  TreatAsAtomicUnit=on
  BPP_faild_ovrd : Constant  Value=0  OutDataTypeStr=boolean
  BrakeFailureDetection : Subsystem
  Bus Creator : BusCreator  Inputs=7
  Bus Selector : BusSelector  OutputSignals=DriverControls_Conv.APP1 [%],DriverControls_Conv.APP2[%],DriverControls_Conv.BPP [%],DriverControls_Conv.V [mph],DriverControls_Conv.keyPos [0_3],DriverControls_Conv.PRNDL
  ClearAPP1fault : Constant  Value=0
  ClearAPP2fault : Constant  Value=0
  Constant2 : Constant  Value=0
  Constant3 : Constant  OutDataTypeStr=boolean
  Conversion  APP1 (%)1 : DataTypeConversion  OutDataTypeStr=boolean
  Conversion  APP1 (%)2 : DataTypeConversion
  Conversion  APP1 (%)3 : DataTypeConversion
  Drv_APP1_valid_ovrd : Constant  Value=0  OutDataTypeStr=boolean
  Drv_APP2_valid_ovrd : Constant  Value=0  OutDataTypeStr=boolean
  Interval Test : simulink/Logic and Bit Operations/Interval Test  IntervalClosedRight=on  uplimit=100  IntervalClosedLeft=on  lowlimit=0  OutDataTypeStr=boolean
  Interval Test1 : simulink/Logic and Bit Operations/Interval Test  IntervalClosedRight=on  uplimit=3  IntervalClosedLeft=on  lowlimit=0  OutDataTypeStr=boolean
  Latch : Subsystem
  Latch1 : Subsystem
  Logical Operator1 : Logic  AllPortsSameDT=off  OutDataTypeStr=boolean
  Logical Operator5 : Logic  Operator=OR  AllPortsSameDT=off  OutDataTypeStr=boolean
  Logical Operator6 : Logic  Operator=OR  AllPortsSameDT=off  OutDataTypeStr=boolean
  PRNDL In range? : simulink/Logic and Bit Operations/Interval Test  IntervalClosedRight=on  uplimit=4  IntervalClosedLeft=on  lowlimit=0  OutDataTypeStr=boolean
  Pulse Generator : DiscretePulseGenerator  PulseType=Time based  Period=0.1  PulseWidth=10
  Scope : Scope
  Driver_SigDiag : Outport
  wires:
  Pulse Generator/1 -> Scope/1, BrakeFailureDetection/Trigger
  BPP_faild_ovrd/1 -> Logical Operator1/1
  Latch1/1(Out1) -> Logical Operator1/2  "Brake_Failed"
  Logical Operator1/1 -> Conversion  APP1 (%)2/1  "Brake_Failed"
  Latch/1(Drv_APP_Agree) -> Conversion  APP1 (%)3/1  "Drv_APP_Agree"
  Interval Test1/1 -> Bus Creator/6  "Drv_KeyPos_[0 3]_SigValid"
  Conversion  APP1 (%)2/1 -> Bus Creator/5  "Brake_Failed"
  Conversion  APP1 (%)3/1 -> Bus Creator/3  "Drv_APP_Agree"
  AccPedalValidity/1(signalValid) -> Logical Operator6/2  "Drv_APP1_[%]_SigValid"
  Drv_APP1_valid_ovrd/1 -> Logical Operator6/1
  AccPedalValidity1/1(signalValid) -> Logical Operator5/2  "Drv_APP2_[%]_SigValid"
  Drv_APP2_valid_ovrd/1 -> Logical Operator5/1
  PRNDL In range?/1 -> Bus Creator/7  "Drv_PRNDL_SigValid"
  BrakeFailureDetection/1(DecelFail) -> Latch1/1(In1)  "Brake_Failed"
  Conversion  APP1 (%)1/1 -> Latch1/2(In2)
  Constant2/1 -> Conversion  APP1 (%)1/1
  Bus Selector/4 -> BrakeFailureDetection/2(VehSpeed)  "<V [mph]>"
  APP_Crosscheck/1(Out1) -> Latch/1(In1)  "Drv_APP_Agree"
  Constant3/1 -> Latch/2(In2)
  Bus Selector/6 -> PRNDL In range?/1  "<PRNDL>"
  Bus Creator/1 -> Driver_SigDiag/1  "Driver_SignalDiag"
  Logical Operator5/1 -> Bus Creator/2  "Drv_APP2_[%]_SigValid"
  Interval Test/1 -> Bus Creator/4  "Drv_BPP_[%]_SigValid"
  Logical Operator6/1 -> Bus Creator/1  "Drv_APP1_[%]_SigValid"
  Bus Selector/5 -> Interval Test1/1  "<keyPos [0_3]>"
  Bus Selector/3 -> BrakeFailureDetection/1(BPP), Interval Test/1  "<BPP [%]>"
  ClearAPP2fault/1 -> AccPedalValidity1/1(clearFaults)
  ClearAPP1fault/1 -> AccPedalValidity/1(clearFaults)
  Bus Selector/2 -> APP_Crosscheck/2(In2), AccPedalValidity1/2(signalValue)  "<APP2[%]>"
  Bus Selector/1 -> APP_Crosscheck/1(In1), AccPedalValidity/2(signalValue)  "<APP1 [%]>"
  Sensors1/1 -> Bus Selector/1
